simulink library "sensor_proc_lib"  (R2016b)
settings: Solver=VariableStepAuto  StartTime=0.0  StopTime=10.0  RelTol=1e-3
undefined symbols (not defined in the file or in its folder): fsw_params
libraries: sensor_processing_libs x4, GPS_processing_lib x1
settings Model: Creator=taylorreynolds  LastModifiedBy=Taylor

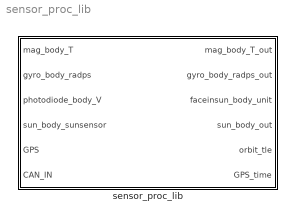
== system sensor_proc_lib ==
  sensor_proc_lib : Subsystem

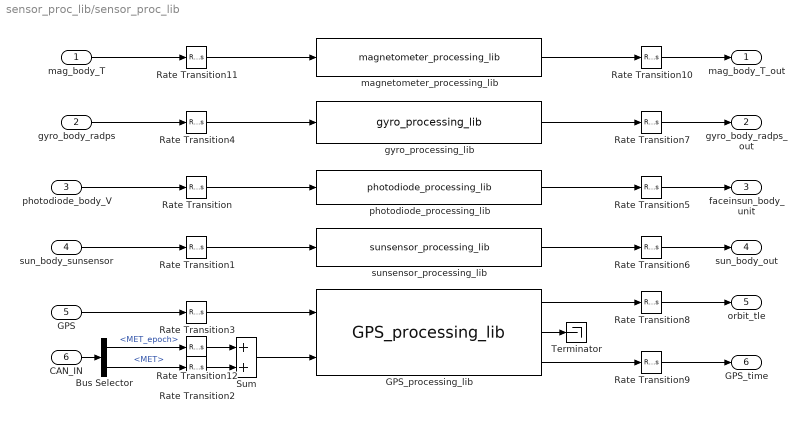
== system sensor_proc_lib/sensor_proc_lib ==
  mag_body_T : Inport
  gyro_body_radps : Inport  Port=2
  photodiode_body_V : Inport  Port=3
  sun_body_sunsensor : Inport  Port=4
  GPS : Inport  Port=5
  CAN_IN : Inport  Port=6
  Bus Selector : BusSelector  OutputSignals=MET_epoch,MET
  GPS_processing_lib : GPS_processing_lib/GPS_processing_lib
  Rate Transition{,1..2,4,11} (5 alike) : RateTransition  OutPortSampleTime=fsw_params.sensor_processing.MSP_SP.sample_time_s
  Rate Transition{5..7,10} (4 alike) : RateTransition
  Rate Transition12 : RateTransition  X0=fsw_params.sensor_processing.gps.JD_J2000_TT_s  OutPortSampleTime=fsw_params.sensor_processing.MSP_SP.sample_time_s
  Rate Transition3 : RateTransition  X0=fsw_params.sensor_processing.gps.ic.all  OutPortSampleTime=fsw_params.sensor_processing.MSP_SP.sample_time_s
  Rate Transition8 : RateTransition  X0=fsw_params.environment.sgp4.orbit_tle
  Rate Transition9 : RateTransition  X0=fsw_params.sensor_processing.gps.ic.time
  Sum : Sum
  Terminator : Terminator
  gyro_processing_lib : sensor_processing_libs/gyro_processing_lib
  magnetometer_processing_lib : sensor_processing_libs/magnetometer_processing_lib
  photodiode_processing_lib : sensor_processing_libs/photodiode_processing_lib
  sunsensor_processing_lib : sensor_processing_libs/sunsensor_processing_lib
  mag_body_T_out : Outport
  gyro_body_radps_out : Outport  Port=2
  faceinsun_body_unit : Outport  Port=3
  sun_body_out : Outport  Port=4
  orbit_tle : Outport  Port=5
  GPS_time : Outport  Port=6
  wires:
  Rate Transition5/1 -> faceinsun_body_unit/1
  photodiode_processing_lib/1 -> Rate Transition5/1
  GPS_processing_lib/3 -> Rate Transition9/1
  GPS_processing_lib/1 -> Rate Transition8/1
  sunsensor_processing_lib/1 -> Rate Transition6/1
  Rate Transition/1 -> photodiode_processing_lib/1
  Rate Transition1/1 -> sunsensor_processing_lib/1
  Rate Transition3/1 -> GPS_processing_lib/1
  GPS_processing_lib/2 -> Terminator/1
  Sum/1 -> GPS_processing_lib/2
  photodiode_body_V/1 -> Rate Transition/1
  CAN_IN/1 -> Bus Selector/1
  GPS/1 -> Rate Transition3/1
  sun_body_sunsensor/1 -> Rate Transition1/1
  Rate Transition9/1 -> GPS_time/1
  Rate Transition8/1 -> orbit_tle/1
  Rate Transition6/1 -> sun_body_out/1
  Bus Selector/1 -> Rate Transition12/1  "<MET_epoch>"
  Bus Selector/2 -> Rate Transition2/1  "<MET>"
  Rate Transition12/1 -> Sum/1
  Rate Transition2/1 -> Sum/2
  gyro_processing_lib/1 -> Rate Transition7/1
  gyro_body_radps/1 -> Rate Transition4/1
  magnetometer_processing_lib/1 -> Rate Transition10/1
  mag_body_T/1 -> Rate Transition11/1
  Rate Transition4/1 -> gyro_processing_lib/1
  Rate Transition7/1 -> gyro_body_radps_out/1
  Rate Transition10/1 -> mag_body_T_out/1
  Rate Transition11/1 -> magnetometer_processing_lib/1
